simulink library "NCS_Library"  (R2019a)
settings: Solver=VariableStepAuto  StartTime=0.0  StopTime=10.0  RelTol=1e-3
values from neighbouring files (symbols this model uses):
  A = 10    [Parameter.m]
  band = 100000000    [Parameter.m]
  BER = 0    [Parameter.m]
  c = 5000000    [Parameter.m]
  c1 = 4.33    [Parameter.m]
  c2 = 3.16    [Parameter.m]
  CAN2EthernetDelay = 0.000    (= 0)    [Parameter.m]
  cR = 1.5*10^-3    (= 0.0015)    [Parameter.m]
  cw = (cwE * 2 + cwM * (nW_ges-2))/nW_ges    (= 0.1475)    [Parameter.m]
  cwE = 0.35    [Parameter.m]
  cwM = 0.08    [Parameter.m]
  Cycle_Controller = 0    [Parameter.m]
  CyclePLC = 24/1000    (= 0.024)    [Parameter.m]
  d = 800000    [Parameter.m]
  Dr = 0.92    [Parameter.m]
  Ethernet2CANDelay = 0.005    [Parameter.m]
  F_konst = 70892    [Parameter.m]
  FA = 100000    [Parameter.m]
  FB_WB_max = 10000    [Parameter.m]
  FBel_an = iG*nG*F_KZmax*nBan*R_mR/(Dr/2)    (= 28197.4297239)    [Parameter.m]
  FBel_frei = iG*nG*F_KZmax*nBfrei*R_mW/(Dr/2)    (= 29270.6882948)    [Parameter.m]
  Fmaxdyn = 300000    [Parameter.m]
  g = 9.81    [Parameter.m]
  i = 0    [Parameter.m]
  J = 1/2*mA*(Dr/2)^2    (= 158.7)    [Parameter.m]
  k1 = 0.095    [Parameter.m]
  k2 = 9.26/3.6    (= 2.57222222222)    [Parameter.m]
  k3 = 4.63/3.6    (= 1.28611111111)    [Parameter.m]
  mges = 58000    [Parameter.m]
  mu = [mu1 mu2]    [Parameter.m]
  muBel1 = 0.42    [Parameter.m]
  muBel2 = 0.36    [Parameter.m]
  n = 0.001    [Parameter.m]
  n_Mg = 4    [Parameter.m]
  n_WB = 4    [Parameter.m]
  nA = 4    [Parameter.m]
  nBan = 2    [Parameter.m]
  nBfrei = 3    [Parameter.m]
  nM = 4    [Parameter.m]
  nW_an = 4    [Parameter.m]
  P_max = 8200000    [Parameter.m]
  Q = 10    [Parameter.m]
  r_reib = 600    [Parameter.m]
  rho = 1.08    [Parameter.m]
  rhoL = 1.225    [Parameter.m]
  Size = 8    [Parameter.m]
  slip = [s1 s2]    [Parameter.m]
  tol = 0.05    [Parameter.m]
  v00 = 100/3.6    (= 27.7777777778)    [Parameter.m]
  v_grenz = 60/3.6    (= 16.6666666667)    [Parameter.m]
  v_opt = 75/3.6    (= 20.8333333333)    [Parameter.m]
  W_opt = 0.5    [Parameter.m]
  WB = 1    [Parameter.m]
  y_opt = sqrt(W_opt)/((1+sqrt(W_opt))^2+W_opt)    [Parameter.m]
undefined symbols (not defined in the file or in its folder): BUSCapacity, CableLength, controlGate, D_dyn, D_mg, EnableBurst, EnableToF, entity, Entity_out, Gate, Gate_4, Gate_5, Gate_ACK, Gate_copy, Gate_RX, getData, gettime, I_dyn, I_mg, m, magnitude, P_dyn, P_mg, ReadAttributes, readdata, ReadData, ReadSize, sigbuilder_block, Timeout, ToB, ToF, v0, v_d, v_soll
libraries: simulink x176, $bdroot x102
(part 2 of 12)

== system NCS_Library/Network/ETB ==
  note: Devices
  note: Bus
  Burst Device : Subsystem  mask{Address=[111 299], Destination=[ 100 200], Size=100, Port=1, ReplyAddress=[0 0], Subscribe=[0 0; 0 0; 0 0; 0 0; 0 0], msgType=Passive, Tx=0, Timeout=0, SDTv2=Disable, EnableToF=off, ToF=0, EnableBurst=off, ToB=0, n_Burst=1000}
      mask prompts: Size "Packet Size [Byte]"; Port "Destination Port"; ReplyAddress "Reply Address"; Tx "Tx [s]"; Timeout "TRDP Timeout [s]"; EnableToF "Enable Failure"; ToF "Time [s]"; EnableBurst "Enable Burst"; ToB "Time [s]"
      mask help: The burst device transmit a user defined number n of useless entities in the network at a user defined time.
      mask init:
      | msgType = uint8(3);
      | Timeout = inf;
      | EnableToF = 0;
      | Tx = 0;
      | % limit n_Burst to 1
      | if n_Burst < 1
      |     n_Burst = 1;
      | end
      mask TypeOptions Port: 1 | 2 | 3 | 4 | 5 | 6 | 7 | 8 | Multicast
      mask TypeOptions msgType: Pull | Push Continuous | Push Discrete | Passive
      mask Callback msgType:
      | % Control parameter visiblity
      | % Disable Tx dialog, if it is not needed, because of a passive ED,
      | % which only receives.
      | 
      | % Get value
      | Modus = get_param(gcb,'msgType');
      | ToF = get_param(gcb,'EnableToF');
      | ToB = get_param(gcb,'EnableBurst');
      | 
      | 
      | % Set the 'MaskVisibilities' property for each box
      | 
      | On = {'on','on','on','on','on','on','on','on','on','on','on','on','on','on','on'}; % Init
      | 
      | % Disable Tx Dialog, if not needed
      | 
      | if strcmp('Passive',Modus) || strcmp('Push Discrete',Modus)
      |     On{8} = 'off';
      | end
      | 
      | if strcmp('off',ToF)
      |     On{12} = 'off';
      | end
      | 
      | if strcmp('off',ToB)
      |     On{14} = 'off';
      |     On{15} = 'off';
      | end
      | 
      | set_param(gcb,'MaskEnables',On );
      mask TypeOptions SDTv2: Disable | Enable
      mask Callback EnableToF:
      | % Control parameter visiblity
      | % Disable Tx dialog, if it is not needed, because of a passive ED,
      | % which only receives.
      | 
      | % Get value
      | Modus = get_param(gcb,'msgType');
      | ToF = get_param(gcb,'EnableToF');
      | ToB = get_param(gcb,'EnableBurst');
      | 
      | 
      | % Set the 'MaskVisibilities' property for each box
      | 
      | On = {'on','on','on','on','on','on','on','on','on','on','on','on','on','on','on'}; % Init
      | 
      | % Disable Tx Dialog, if not needed
      | 
      | if strcmp('Passive',Modus) || strcmp('Push Discrete',Modus)
      |     On{8} = 'off';
      | end
      | 
      | if strcmp('off',ToF)
      |     On{12} = 'off';
      | end
      | 
      | if strcmp('off',ToB)
      |     On{14} = 'off';
      |     On{15} = 'off';
      | end
      | 
      | set_param(gcb,'MaskEnables',On );
      mask Callback EnableBurst:
      | % Control parameter visiblity
      | % Disable Tx dialog, if it is not needed, because of a passive ED,
      | % which only receives.
      | 
      | % Get value
      | Modus = get_param(gcb,'msgType');
      | ToF = get_param(gcb,'EnableToF');
      | ToB = get_param(gcb,'EnableBurst');
      | 
      | 
      | % Set the 'MaskVisibilities' property for each box
      | 
      | On = {'on','on','on','on','on','on','on','on','on','on','on','on','on','on','on'}; % Init
      | 
      | % Disable Tx Dialog, if not needed
      | 
      | if strcmp('Passive',Modus) || strcmp('Push Discrete',Modus)
      |     On{8} = 'off';
      | end
      | 
      | if strcmp('off',ToF)
      |     On{12} = 'off';
      | end
      | 
      | if strcmp('off',ToB)
      |     On{14} = 'off';
      |     On{15} = 'off';
      | end
      | 
      | set_param(gcb,'MaskEnables',On );
      mask DialogControl Container3 Prompt: Modus
      mask DialogControl Container4 Prompt: SDTv2
      mask DialogControl Container6 Prompt: Interrupts
      mask Display: disp([ 'Burst Device' ]);
  Cable : Subsystem  mask{length=0, Cable=Coaxial}
      mask prompts: length "Cable Length (m)"; Cable "Cable Type"
      mask TypeOptions Cable: Coaxial | Other
  Controller Interface : Subsystem  mask{Address=[111 211], Sensors=[0 0; 0 0; 0 0; 0 0], Actuators=[0 0; 0 0; 0 0; 0 0], Size=11, EnableToF=off, ToF=0, Enable_1=off, msgType_1=Push by Controller, SDTv2_1=Disable, Tx_1=0, Enable_2=off, msgType_2=Push by Controller, SDTv2_2=Disable, Tx_2=0, Enable_3=off, msgType_3=Push by Controller, SDTv2_3=Disable, Tx_3=0, Enable_4=off, msgType_4=Push by Controller, SDTv2_4=Disable, Tx_4=0}
      mask prompts: Size "Packet Size [Byte]"; EnableToF "Failure"; ToF "Time [s]"; Enable_1 "Enable"; msgType_1 "Modus"; SDTv2_1 "SDTv2"; Tx_1 "Tx [ms]"; Enable_2 "Enable"; msgType_2 "Modus"; SDTv2_2 "SDTv2"; Tx_2 "Tx [ms]"; Enable_3 "Enable"; msgType_3 "Modus"; SDTv2_3 "SDTv2"; Tx_3 "Tx [ms]"; Enable_4 "Enable"; msgType_4 "Modus"; SDTv2_4 "SDTv2"; Tx_4 "Tx [ms]"
      mask help: Tx can be set to zero in case of a discrete source
      mask init:
      | % Ensure, that Tx is set to zero in the case of pull.
      | if msgType_1 == 2 || ~Enable_1
      |     Tx_1 = inf;
      | else
      |     % convert [ms] to [s]
      |     Tx_1 = Tx_1/1000;
      | end
      | 
      | if msgType_2 == 2 || ~Enable_2
      |     Tx_2 = inf;
      | else
      |     % convert [ms] to [s]
      |     Tx_2 = Tx_2/1000;
      | end
      | 
      | if msgType_3 == 2 || ~Enable_3
      |     Tx_3 = inf;
      | else
      |     % convert [ms] to [s]
      |     Tx_3 = Tx_3/1000;
      | end
      | 
      | if msgType_4 == 2 || ~Enable_4
      |     Tx_4 = inf;
      | else
      |     % convert [ms] to [s]
      |     Tx_4 = Tx_4/1000;
      | end
      | 
      | % 
      | if ~Enable_1 && ~Enable_2 && ~Enable_3 && ~Enable_4
      |     Actuators = zeros(4,2);
      | end
      mask Callback EnableToF:
      | % Control parameter visiblity
      | 
      | % Get the values of the Modus boxes
      | Enable_1 = get_param(gcb,'Enable_1');
      | Enable_2 = get_param(gcb,'Enable_2');
      | Enable_3 = get_param(gcb,'Enable_3');
      | Enable_4 = get_param(gcb,'Enable_4');
      | 
      | Modus_1 = get_param(gcb,'msgType_1');
      | Modus_2 = get_param(gcb,'msgType_2');
      | Modus_3 = get_param(gcb,'msgType_3');
      | Modus_4 = get_param(gcb,'msgType_4');
      | 
      | EnableToF = get_param(gcb,'EnableToF');
      | 
      | % Set the 'MaskVisibilities' property for each box
      | 
      | On = {'on','on','on','on','on','on','on','on','on','on','on','on','on','on','on','on','on','on','on','on','on','on'}; % Init
      | 
      | % Disable Port Dialog, if not needed
      | if strcmp('off',Enable_1)
      |     On{7} = 'off';
      |     On{8} = 'off';
      |     On{9} = 'off';
      | end
      | if strcmp('off',Enable_2)
      |     On{11} = 'off';
      |     On{12} = 'off';
      |     On{13} = 'off';
      | end
      | if strcmp('off',Enable_3)
      |     On{15} = 'off';
      |     On{16} = 'off';
      |     On{17} = 'off';
      | end
      | if strcmp('off',Enable_4)
      |     On{19} = 'off';
      |     On{20} = 'off';
      |     On{21} = 'off';
      | end
      | 
      | % Disable Tx Dialog, if not needed
      | 
      | if ~strcmp('Push by Controller',Modus_1)
      |     On{9} = 'off';
      | end
      | if ~strcmp('Push by Controller',Modus_2)
      |     On{13} = 'off';
      | end
      | if ~strcmp('Push by Controller',Modus_3)
      |     On{17} = 'off';
      | end
      | if ~strcmp('Push by Controller',Modus_4)
      |     On{21} = 'off';
      | end
      | 
      | if strcmp('off',EnableToF)
      |     On{5} = 'off';
      | end
      | 
      | set_param(gcb,'MaskEnables',On );
      mask Callback Enable_1:
      | % Control parameter visiblity
      | 
      | % Get the values of the Modus boxes
      | Enable_1 = get_param(gcb,'Enable_1');
      | Enable_2 = get_param(gcb,'Enable_2');
      | Enable_3 = get_param(gcb,'Enable_3');
      | Enable_4 = get_param(gcb,'Enable_4');
      | 
      | Modus_1 = get_param(gcb,'msgType_1');
      | Modus_2 = get_param(gcb,'msgType_2');
      | Modus_3 = get_param(gcb,'msgType_3');
      | Modus_4 = get_param(gcb,'msgType_4');
      | 
      | EnableToF = get_param(gcb,'EnableToF');
      | 
      | % Set the 'MaskVisibilities' property for each box
      | 
      | On = {'on','on','on','on','on','on','on','on','on','on','on','on','on','on','on','on','on','on','on','on','on','on'}; % Init
      | 
      | % Disable Port Dialog, if not needed
      | if strcmp('off',Enable_1)
      |     On{7} = 'off';
      |     On{8} = 'off';
      |     On{9} = 'off';
      | end
      | if strcmp('off',Enable_2)
      |     On{11} = 'off';
      |     On{12} = 'off';
      |     On{13} = 'off';
      | end
      | if strcmp('off',Enable_3)
      |     On{15} = 'off';
      |     On{16} = 'off';
      |     On{17} = 'off';
      | end
      | if strcmp('off',Enable_4)
      |     On{19} = 'off';
      |     On{20} = 'off';
      |     On{21} = 'off';
      | end
      | 
      | % Disable Tx Dialog, if not needed
      | 
      | if ~strcmp('Push by Controller',Modus_1)
      |     On{9} = 'off';
      | end
      | if ~strcmp('Push by Controller',Modus_2)
      |     On{13} = 'off';
      | end
      | if ~strcmp('Push by Controller',Modus_3)
      |     On{17} = 'off';
      | end
      | if ~strcmp('Push by Controller',Modus_4)
      |     On{21} = 'off';
      | end
      | 
      | if strcmp('off',EnableToF)
      |     On{5} = 'off';
      | end
      | 
      | set_param(gcb,'MaskEnables',On );
      mask TypeOptions msgType_1: Push by Controller | Pull by Actuator
      mask Callback msgType_1:
      | % Control parameter visiblity
      | 
      | % Get the values of the Modus boxes
      | Enable_1 = get_param(gcb,'Enable_1');
      | Enable_2 = get_param(gcb,'Enable_2');
      | Enable_3 = get_param(gcb,'Enable_3');
      | Enable_4 = get_param(gcb,'Enable_4');
      | 
      | Modus_1 = get_param(gcb,'msgType_1');
      | Modus_2 = get_param(gcb,'msgType_2');
      | Modus_3 = get_param(gcb,'msgType_3');
      | Modus_4 = get_param(gcb,'msgType_4');
      | 
      | EnableToF = get_param(gcb,'EnableToF');
      | 
      | % Set the 'MaskVisibilities' property for each box
      | 
      | On = {'on','on','on','on','on','on','on','on','on','on','on','on','on','on','on','on','on','on','on','on','on','on'}; % Init
      | 
      | % Disable Port Dialog, if not needed
      | if strcmp('off',Enable_1)
      |     On{7} = 'off';
      |     On{8} = 'off';
      |     On{9} = 'off';
      | end
      | if strcmp('off',Enable_2)
      |     On{11} = 'off';
      |     On{12} = 'off';
      |     On{13} = 'off';
      | end
      | if strcmp('off',Enable_3)
      |     On{15} = 'off';
      |     On{16} = 'off';
      |     On{17} = 'off';
      | end
      | if strcmp('off',Enable_4)
      |     On{19} = 'off';
      |     On{20} = 'off';
      |     On{21} = 'off';
      | end
      | 
      | % Disable Tx Dialog, if not needed
      | 
      | if ~strcmp('Push by Controller',Modus_1)
      |     On{9} = 'off';
      | end
      | if ~strcmp('Push by Controller',Modus_2)
      |     On{13} = 'off';
      | end
      | if ~strcmp('Push by Controller',Modus_3)
      |     On{17} = 'off';
      | end
      | if ~strcmp('Push by Controller',Modus_4)
      |     On{21} = 'off';
      | end
      | 
      | if strcmp('off',EnableToF)
      |     On{5} = 'off';
      | end
      | 
      | set_param(gcb,'MaskEnables',On );
      mask TypeOptions SDTv2_1: Disable | Enable
      mask Callback Enable_2:
      | % Control parameter visiblity
      | 
      | % Get the values of the Modus boxes
      | Enable_1 = get_param(gcb,'Enable_1');
      | Enable_2 = get_param(gcb,'Enable_2');
      | Enable_3 = get_param(gcb,'Enable_3');
      | Enable_4 = get_param(gcb,'Enable_4');
      | 
      | Modus_1 = get_param(gcb,'msgType_1');
      | Modus_2 = get_param(gcb,'msgType_2');
      | Modus_3 = get_param(gcb,'msgType_3');
      | Modus_4 = get_param(gcb,'msgType_4');
      | 
      | EnableToF = get_param(gcb,'EnableToF');
      | 
      | % Set the 'MaskVisibilities' property for each box
      | 
      | On = {'on','on','on','on','on','on','on','on','on','on','on','on','on','on','on','on','on','on','on','on','on','on'}; % Init
      | 
      | % Disable Port Dialog, if not needed
      | if strcmp('off',Enable_1)
      |     On{7} = 'off';
      |     On{8} = 'off';
      |     On{9} = 'off';
      | end
      | if strcmp('off',Enable_2)
      |     On{11} = 'off';
      |     On{12} = 'off';
      |     On{13} = 'off';
      | end
      | if strcmp('off',Enable_3)
      |     On{15} = 'off';
      |     On{16} = 'off';
      |     On{17} = 'off';
      | end
      | if strcmp('off',Enable_4)
      |     On{19} = 'off';
      |     On{20} = 'off';
      |     On{21} = 'off';
      | end
      | 
      | % Disable Tx Dialog, if not needed
      | 
      | if ~strcmp('Push by Controller',Modus_1)
      |     On{9} = 'off';
      | end
      | if ~strcmp('Push by Controller',Modus_2)
      |     On{13} = 'off';
      | end
      | if ~strcmp('Push by Controller',Modus_3)
      |     On{17} = 'off';
      | end
      | if ~strcmp('Push by Controller',Modus_4)
      |     On{21} = 'off';
      | end
      | 
      | if strcmp('off',EnableToF)
      |     On{5} = 'off';
      | end
      | 
      | set_param(gcb,'MaskEnables',On );
      mask TypeOptions msgType_2: Push by Controller | Pull by Actuator
      mask Callback msgType_2:
      | % Control parameter visiblity
      | 
      | % Get the values of the Modus boxes
      | Enable_1 = get_param(gcb,'Enable_1');
      | Enable_2 = get_param(gcb,'Enable_2');
      | Enable_3 = get_param(gcb,'Enable_3');
      | Enable_4 = get_param(gcb,'Enable_4');
      | 
      | Modus_1 = get_param(gcb,'msgType_1');
      | Modus_2 = get_param(gcb,'msgType_2');
      | Modus_3 = get_param(gcb,'msgType_3');
      | Modus_4 = get_param(gcb,'msgType_4');
      | 
      | EnableToF = get_param(gcb,'EnableToF');
      | 
      | % Set the 'MaskVisibilities' property for each box
      | 
      | On = {'on','on','on','on','on','on','on','on','on','on','on','on','on','on','on','on','on','on','on','on','on','on'}; % Init
      | 
      | % Disable Port Dialog, if not needed
      | if strcmp('off',Enable_1)
      |     On{7} = 'off';
      |     On{8} = 'off';
      |     On{9} = 'off';
      | end
      | if strcmp('off',Enable_2)
      |     On{11} = 'off';
      |     On{12} = 'off';
      |     On{13} = 'off';
      | end
      | if strcmp('off',Enable_3)
      |     On{15} = 'off';
      |     On{16} = 'off';
      |     On{17} = 'off';
      | end
      | if strcmp('off',Enable_4)
      |     On{19} = 'off';
      |     On{20} = 'off';
      |     On{21} = 'off';
      | end
      | 
      | % Disable Tx Dialog, if not needed
      | 
      | if ~strcmp('Push by Controller',Modus_1)
      |     On{9} = 'off';
      | end
      | if ~strcmp('Push by Controller',Modus_2)
      |     On{13} = 'off';
      | end
      | if ~strcmp('Push by Controller',Modus_3)
      |     On{17} = 'off';
      | end
      | if ~strcmp('Push by Controller',Modus_4)
      |     On{21} = 'off';
      | end
      | 
      | if strcmp('off',EnableToF)
      |     On{5} = 'off';
      | end
      | 
      | set_param(gcb,'MaskEnables',On );
      mask TypeOptions SDTv2_2: Disable | Enable
      mask Callback Enable_3:
      | % Control parameter visiblity
      | 
      | % Get the values of the Modus boxes
      | Enable_1 = get_param(gcb,'Enable_1');
      | Enable_2 = get_param(gcb,'Enable_2');
      | Enable_3 = get_param(gcb,'Enable_3');
      | Enable_4 = get_param(gcb,'Enable_4');
      | 
      | Modus_1 = get_param(gcb,'msgType_1');
      | Modus_2 = get_param(gcb,'msgType_2');
      | Modus_3 = get_param(gcb,'msgType_3');
      | Modus_4 = get_param(gcb,'msgType_4');
      | 
      | EnableToF = get_param(gcb,'EnableToF');
      | 
      | % Set the 'MaskVisibilities' property for each box
      | 
      | On = {'on','on','on','on','on','on','on','on','on','on','on','on','on','on','on','on','on','on','on','on','on','on'}; % Init
      | 
      | % Disable Port Dialog, if not needed
      | if strcmp('off',Enable_1)
      |     On{7} = 'off';
      |     On{8} = 'off';
      |     On{9} = 'off';
      | end
      | if strcmp('off',Enable_2)
      |     On{11} = 'off';
      |     On{12} = 'off';
      |     On{13} = 'off';
      | end
      | if strcmp('off',Enable_3)
      |     On{15} = 'off';
      |     On{16} = 'off';
      |     On{17} = 'off';
      | end
      | if strcmp('off',Enable_4)
      |     On{19} = 'off';
      |     On{20} = 'off';
      |     On{21} = 'off';
      | end
      | 
      | % Disable Tx Dialog, if not needed
      | 
      | if ~strcmp('Push by Controller',Modus_1)
      |     On{9} = 'off';
      | end
      | if ~strcmp('Push by Controller',Modus_2)
      |     On{13} = 'off';
      | end
      | if ~strcmp('Push by Controller',Modus_3)
      |     On{17} = 'off';
      | end
      | if ~strcmp('Push by Controller',Modus_4)
      |     On{21} = 'off';
      | end
      | 
      | if strcmp('off',EnableToF)
      |     On{5} = 'off';
      | end
      | 
      | set_param(gcb,'MaskEnables',On );
      mask TypeOptions msgType_3: Push by Controller | Pull by Actuator
      mask Callback msgType_3:
      | % Control parameter visiblity
      | 
      | % Get the values of the Modus boxes
      | Enable_1 = get_param(gcb,'Enable_1');
      | Enable_2 = get_param(gcb,'Enable_2');
      | Enable_3 = get_param(gcb,'Enable_3');
      | Enable_4 = get_param(gcb,'Enable_4');
      | 
      | Modus_1 = get_param(gcb,'msgType_1');
      | Modus_2 = get_param(gcb,'msgType_2');
      | Modus_3 = get_param(gcb,'msgType_3');
      | Modus_4 = get_param(gcb,'msgType_4');
      | 
      | EnableToF = get_param(gcb,'EnableToF');
      | 
      | % Set the 'MaskVisibilities' property for each box
      | 
      | On = {'on','on','on','on','on','on','on','on','on','on','on','on','on','on','on','on','on','on','on','on','on','on'}; % Init
      | 
      | % Disable Port Dialog, if not needed
      | if strcmp('off',Enable_1)
      |     On{7} = 'off';
      |     On{8} = 'off';
      |     On{9} = 'off';
      | end
      | if strcmp('off',Enable_2)
      |     On{11} = 'off';
      |     On{12} = 'off';
      |     On{13} = 'off';
      | end
      | if strcmp('off',Enable_3)
      |     On{15} = 'off';
      |     On{16} = 'off';
      |     On{17} = 'off';
      | end
      | if strcmp('off',Enable_4)
      |     On{19} = 'off';
      |     On{20} = 'off';
      |     On{21} = 'off';
      | end
      | 
      | % Disable Tx Dialog, if not needed
      | 
      | if ~strcmp('Push by Controller',Modus_1)
      |     On{9} = 'off';
      | end
      | if ~strcmp('Push by Controller',Modus_2)
      |     On{13} = 'off';
      | end
      | if ~strcmp('Push by Controller',Modus_3)
      |     On{17} = 'off';
      | end
      | if ~strcmp('Push by Controller',Modus_4)
      |     On{21} = 'off';
      | end
      | 
      | if strcmp('off',EnableToF)
      |     On{5} = 'off';
      | end
      | 
      | set_param(gcb,'MaskEnables',On );
      mask TypeOptions SDTv2_3: Disable | Enable
      mask Callback Enable_4:
      | % Control parameter visiblity
      | 
      | % Get the values of the Modus boxes
      | Enable_1 = get_param(gcb,'Enable_1');
      | Enable_2 = get_param(gcb,'Enable_2');
      | Enable_3 = get_param(gcb,'Enable_3');
      | Enable_4 = get_param(gcb,'Enable_4');
      | 
      | Modus_1 = get_param(gcb,'msgType_1');
      | Modus_2 = get_param(gcb,'msgType_2');
      | Modus_3 = get_param(gcb,'msgType_3');
      | Modus_4 = get_param(gcb,'msgType_4');
      | 
      | EnableToF = get_param(gcb,'EnableToF');
      | 
      | % Set the 'MaskVisibilities' property for each box
      | 
      | On = {'on','on','on','on','on','on','on','on','on','on','on','on','on','on','on','on','on','on','on','on','on','on'}; % Init
      | 
      | % Disable Port Dialog, if not needed
      | if strcmp('off',Enable_1)
      |     On{7} = 'off';
      |     On{8} = 'off';
      |     On{9} = 'off';
      | end
      | if strcmp('off',Enable_2)
      |     On{11} = 'off';
      |     On{12} = 'off';
      |     On{13} = 'off';
      | end
      | if strcmp('off',Enable_3)
      |     On{15} = 'off';
      |     On{16} = 'off';
      |     On{17} = 'off';
      | end
      | if strcmp('off',Enable_4)
      |     On{19} = 'off';
      |     On{20} = 'off';
      |     On{21} = 'off';
      | end
      | 
      | % Disable Tx Dialog, if not needed
      | 
      | if ~strcmp('Push by Controller',Modus_1)
      |     On{9} = 'off';
      | end
      | if ~strcmp('Push by Controller',Modus_2)
      |     On{13} = 'off';
      | end
      | if ~strcmp('Push by Controller',Modus_3)
      |     On{17} = 'off';
      | end
      | if ~strcmp('Push by Controller',Modus_4)
      |     On{21} = 'off';
      | end
      | 
      | if strcmp('off',EnableToF)
      |     On{5} = 'off';
      | end
      | 
      | set_param(gcb,'MaskEnables',On );
      mask TypeOptions msgType_4: Push by Controller | Pull by Actuator
      mask Callback msgType_4:
      | % Control parameter visiblity
      | 
      | % Get the values of the Modus boxes
      | Enable_1 = get_param(gcb,'Enable_1');
      | Enable_2 = get_param(gcb,'Enable_2');
      | Enable_3 = get_param(gcb,'Enable_3');
      | Enable_4 = get_param(gcb,'Enable_4');
      | 
      | Modus_1 = get_param(gcb,'msgType_1');
      | Modus_2 = get_param(gcb,'msgType_2');
      | Modus_3 = get_param(gcb,'msgType_3');
      | Modus_4 = get_param(gcb,'msgType_4');
      | 
      | EnableToF = get_param(gcb,'EnableToF');
      | 
      | % Set the 'MaskVisibilities' property for each box
      | 
      | On = {'on','on','on','on','on','on','on','on','on','on','on','on','on','on','on','on','on','on','on','on','on','on'}; % Init
      | 
      | % Disable Port Dialog, if not needed
      | if strcmp('off',Enable_1)
      |     On{7} = 'off';
      |     On{8} = 'off';
      |     On{9} = 'off';
      | end
      | if strcmp('off',Enable_2)
      |     On{11} = 'off';
      |     On{12} = 'off';
      |     On{13} = 'off';
      | end
      | if strcmp('off',Enable_3)
      |     On{15} = 'off';
      |     On{16} = 'off';
      |     On{17} = 'off';
      | end
      | if strcmp('off',Enable_4)
      |     On{19} = 'off';
      |     On{20} = 'off';
      |     On{21} = 'off';
      | end
      | 
      | % Disable Tx Dialog, if not needed
      | 
      | if ~strcmp('Push by Controller',Modus_1)
      |     On{9} = 'off';
      | end
      | if ~strcmp('Push by Controller',Modus_2)
      |     On{13} = 'off';
      | end
      | if ~strcmp('Push by Controller',Modus_3)
      |     On{17} = 'off';
      | end
      | if ~strcmp('Push by Controller',Modus_4)
      |     On{21} = 'off';
      | end
      | 
      | if strcmp('off',EnableToF)
      |     On{5} = 'off';
      | end
      | 
      | set_param(gcb,'MaskEnables',On );
      mask TypeOptions SDTv2_4: Disable | Enable
      mask DialogControl Container13 Prompt: Interrupt
      mask DialogControl Container9 Prompt: Port 1
      mask DialogControl Container10 Prompt: Port 2
      mask DialogControl Container11 Prompt: Port 3
      mask DialogControl Container12 Prompt: Port 4
      mask Display: disp([ 'Ethernet \n Controller Interface' '\n' get_param(gcb,'Address') ]);
  ED : Subsystem  mask{Address=[111 211], Destination=[ 0 0], Port=1, ReplyAddress=[0 0], Size=11, Subscribe=[0 0; 0 0; 0 0; 0 0; 0 0], msgType=Passive, Tx=0, Timeout=2, SDTv2=Disable, EnableToF=off, ToF=0}
      mask prompts: Port "Destination Port"; ReplyAddress "Reply Address"; Size "Packet Size [Byte]"; Tx "Tx [ms]"; Timeout "TRDP Timeout [s]"; EnableToF "Enable Failure"; ToF "Time [s]"
      mask init:
      | if msgType == 3 || msgType == 4
      |     Tx = 0;
      | else
      |     Tx = Tx/1000;
      | end
      mask TypeOptions Port: 1 | 2 | 3 | 4 | 5 | 6 | 7 | 8 | Multicast
      mask TypeOptions msgType: Pull | Push cyclical | Push sporadic | Passive
      mask Callback msgType:
      | % Control parameter visiblity
      | % Disable Tx dialog, if it is not needed, because of a passive ED,
      | % which only receives.
      | 
      | % Get value
      | Modus = get_param(gcb,'msgType');
      | ToF = get_param(gcb,'EnableToF');
      | 
      | % Set the 'MaskVisibilities' property for each box
      | 
      | On = {'on','on','on','on','on','on','on','on','on','on','on','on'}; % Init
      | 
      | % Disable Tx Dialog, if not needed
      | 
      | if strcmp('Passive',Modus) || strcmp('Push Discrete',Modus)
      |     On{8} = 'off';
      | end
      | 
      | if strcmp('off',ToF)
      |     On{12} = 'off';
      | end
      | 
      | set_param(gcb,'MaskEnables',On );
      mask TypeOptions SDTv2: Disable | Enable
      mask Callback EnableToF:
      | % Control parameter visiblity
      | % Disable Tx dialog, if it is not needed, because of a passive ED,
      | % which only receives.
      | 
      | % Get value
      | Modus = get_param(gcb,'msgType');
      | ToF = get_param(gcb,'EnableToF');
      | 
      | % Set the 'MaskVisibilities' property for each box
      | 
      | On = {'on','on','on','on','on','on','on','on','on','on','on','on'}; % Init
      | 
      | % Disable Tx Dialog, if not needed
      | 
      | if strcmp('Passive',Modus) || strcmp('Push Discrete',Modus)
      |     On{8} = 'off';
      | end
      | 
      | if strcmp('off',ToF)
      |     On{12} = 'off';
      | end
      | 
      | set_param(gcb,'MaskEnables',On );
      mask DialogControl Container3 Prompt: Modus
      mask DialogControl Container4 Prompt: SDTv2
      mask DialogControl Container6 Prompt: Interrupts
      mask Display: disp([ 'End Device' '\n' get_param(gcb,'Address') ]);
  Ethernet_2-port_Switch : Subsystem  mask{addstore=10, bandc=10^8, buffer_size=120000, cable_node=0, cable_LR=0}
      mask prompts: addstore "Number of Addresses to Store on each Port"; bandc "Bandwidth for Switch [bits/s]"; buffer_size "Total Buffer size [bits]"; cable_node "Length of Cable to Node [m]"; cable_LR "Length of Cable to L or R [m]"
      mask init:
      | % band = eval(band);
      mask TypeOptions bandc: 10^7 | 10^8 | 10^9
      mask DialogControl DescGroupVar Prompt: Ethernet 2-Port Switch
      mask DialogControl DescTextVar Prompt: Ethernet Switch with Two Ports, for use at the end of the network.
  Ethernet_3-port_switch : Subsystem  mask{addstore=5, bandc=10^8, buffer_size=180000, cable_node=0, cable_L=0, cable_R=0}
      mask prompts: addstore "Number of addresses to Store on each port"; bandc "Bandwidth of switch [bits/s]"; buffer_size "Total Buffer Size [bits]"; cable_node "Cable length to Node"; cable_L "Cable length to L"; cable_R "Cable length to R"
      mask init:
      | %band = eval(band);
      mask TypeOptions bandc: 10^7 | 10^8 | 10^9
      mask DialogControl DescGroupVar Prompt: Ethernet Switch 3 Ports
      mask DialogControl DescTextVar Prompt: Ethernet Switch with 3 Ports, for use between other switches or nodes within a network.
  OSI Layers : Subsystem
  Subsystem2 : Subsystem  mask{RouterID=1, SubnetIDa=0, SubnetIDb=0, SubnetIDc=0, CycleTime_Router=0.05, EnableToF=off, ToF=0}
      mask prompts: SubnetIDa "1. Subnet"; SubnetIDb "2. Subnet"; SubnetIDc "3. Subnet"; CycleTime_Router "CycleTime"; EnableToF "Failure"; ToF "Time of Failure [s]"
      mask Callback EnableToF:
      | % Control parameter visiblity
      | 
      | % Get value
      | ToF = get_param(gcb,'EnableToF');
      | 
      | 
      | % Set the 'MaskVisibilities' property for each box
      | 
      | On = {'on','on','on','on','on','on','on'}; % Init
      | 
      | % Disable Time Dialog, if not needed
      | if strcmp('off',ToF)
      |     On{7} = 'off';
      | end
      | 
      | set_param(gcb,'MaskEnables',On );
      mask DialogControl Container4 Prompt: Interrupt
      mask Display: disp([ 'Router' '\n ID: '  get_param(gcb,'RouterID') ]);
  Termination : Subsystem

== system NCS_Library/Network/Gateway ==
  note: CAN 1
  note: CAN 2
  Gateway1 : Subsystem  mask{T_Tx=4, MaxNum=20, Address=[111 211], Destination=[0 0], Port=1, ReplyAddress=[0 0], Subscribe=[0 0; 0 0; 0 0; 0 0; 0 0], Timeout=inf, SDTv2=Disable, SensorType=0, MsgID=25, IDRange=[1:25], T_Tx_CAN=0.1, MsgSize=8, IDSubscription=[0,0,0,0,0,0,0,0,0,0,0,0,0,0,0,0,0,0,0,0,0,0,0,0,0], EnableToF=off, ToF=0}
      mask prompts: Port "Destination Port"; ReplyAddress "Reply Address"; MsgID "CAN ID"; IDRange "Range of all IDs"; T_Tx_CAN "T_Tx"; MsgSize "DataSIze (0-8 Bytes)"; IDSubscription "IDs of messages subscribed to accept (0-no, 1-yes)"; EnableToF "Failure"; ToF "Time [s]"
      mask TypeOptions Port: 1 | 2 | 3 | 4 | 5 | 6 | 7 | 8 | Multicast
      mask TypeOptions SDTv2: Disable | Enable
      mask Callback EnableToF:
      | % Control parameter visiblity
      | % Disable Tx dialog, if it is not needed, because of a passive ED,
      | % which only receives.
      | 
      | % Get value
      | ToF = get_param(gcb,'EnableToF');
      | % ToB = get_param(gcb,'EnableBurst');
      | 
      | 
      | % Set the 'MaskVisibilities' property for each box
      | 
      | On = {'on','on','on','on','on','on','on','on','on','on','on','on','on','on','on','on','on'}; % Init
      | 
      | % Disable Tx Dialog, if not needed
      | if strcmp('off',ToF)
      |     On{17} = 'off';
      | end
      | 
      | set_param(gcb,'MaskEnables',On );
      mask DialogControl ParameterGroupVar Prompt: Parameters Gateway
      mask DialogControl Container5 Prompt: Parameters Ethernet Interface
      mask DialogControl Container6 Prompt: SDTv2
      mask DialogControl Container3 Prompt: Paramters CAN Interface
      mask DialogControl Container4 Prompt: Interupts
      mask Display: disp( ['Address: ', get_param(gcb,'Address'), '\n \n Ethernet-CAN-Gateway', '\n \n CAN-ID: ', get_param(gcb,'msgID')] )
  Gateway2 : Subsystem  mask{T_Tx=4, MaxNum=20, Address=[111 211], Destination=[0 0], Port=1, ReplyAddress=[0 0], Subscribe=[0 0; 0 0; 0 0; 0 0; 0 0], Timeout=inf, SDTv2=Disable, SensorType=0, MsgID=25, IDRange=[1:25], T_Tx_CAN=0.1, MsgSize=8, IDSubscription=[0,0,0,0,0,0,0,0,0,0,0,0,0,0,0,0,0,0,0,0,0,0,0,0,0], EnableToF=off, ToF=0}
      mask prompts: Port "Destination Port"; ReplyAddress "Reply Address"; MsgID "CAN ID"; IDRange "Range of all IDs"; T_Tx_CAN "T_Tx"; MsgSize "DataSIze (0-8 Bytes)"; IDSubscription "IDs of messages subscribed to accept (0-no, 1-yes)"; EnableToF "Failure"; ToF "Time [s]"
      mask TypeOptions Port: 1 | 2 | 3 | 4 | 5 | 6 | 7 | 8 | Multicast
      mask TypeOptions SDTv2: Disable | Enable
      mask Callback EnableToF:
      | % Control parameter visiblity
      | % Disable Tx dialog, if it is not needed, because of a passive ED,
      | % which only receives.
      | 
      | % Get value
      | ToF = get_param(gcb,'EnableToF');
      | % ToB = get_param(gcb,'EnableBurst');
      | 
      | 
      | % Set the 'MaskVisibilities' property for each box
      | 
      | On = {'on','on','on','on','on','on','on','on','on','on','on','on','on','on','on','on','on'}; % Init
      | 
      | % Disable Tx Dialog, if not needed
      | if strcmp('off',ToF)
      |     On{17} = 'off';
      | end
      | 
      | set_param(gcb,'MaskEnables',On );
      mask DialogControl ParameterGroupVar Prompt: Parameters Gateway
      mask DialogControl Container5 Prompt: Parameters Ethernet Interface
      mask DialogControl Container6 Prompt: SDTv2
      mask DialogControl Container3 Prompt: Paramters CAN Interface
      mask DialogControl Container4 Prompt: Interupts
      mask Display: disp( ['Address: ', get_param(gcb,'Address'), '\n \n Ethernet-CAN-Gateway', '\n \n CAN-ID: ', get_param(gcb,'msgID')] )

== system NCS_Library/Plant (Train)/Angetriebene_Achse ==
  note: Elektromotor
  note: F_t
  note: Schlupf
  fSt_dyn : Inport
  fSt Achse : Inport  Port=2
  Wagengeschwindigkeit : Inport  Port=3
  1/I : Gain  Gain=1/J  SaturateOnIntegerOverflow=on  OutDataTypeStr=Inherit: Same as input  ParamDataTypeStr=Inherit: Same as input
  Add : Sum  Inputs=-+
  Bremskraft pro angetriebener Achse2 : Subsystem
  Bus Creator : BusCreator  Inputs=3
  Display{,1..6} (7 alike) : Display
  Gain : Gain  Gain=1/1000
  Gain1 : Gain  Gain=1/(Dr/2)  SaturateOnIntegerOverflow=on  OutDataTypeStr=Inherit: Same as input  ParamDataTypeStr=Inherit: Same as input
  Gain2 : Gain
  Kraftschlussbeiwert : Scope
  Max : MinMax  Function=max  Inputs=2
  Neigung : Constant  Value=i
  Product : Product  Inputs=3
  Rad- geschwindigkeit : Integrator  InitialCondition=v0/(Dr/2)  LimitOutput=on  UpperSaturationLimit=1000  LowerSaturationLimit=0
  Radradius : Gain  Gain=Dr/2  SaturateOnIntegerOverflow=on  OutDataTypeStr=Inherit: Same as input  ParamDataTypeStr=Inherit: Same as input
  Radradius1 : Gain  Gain=Dr/2  SaturateOnIntegerOverflow=on  OutDataTypeStr=Inherit: Same as input  ParamDataTypeStr=Inherit: Same as input
  Radradius2 : Gain  Gain=Dr/2  SaturateOnIntegerOverflow=on  OutDataTypeStr=Inherit: Same as input  ParamDataTypeStr=Inherit: Same as input
  Schlupf : Fcn  Expr=abs(u(2)-u(1))/u(3)
  Schlupf-Kraftschluss- Beziehung : Lookup_n-D  NumberOfTableDimensions=1  BreakpointsForDimension1=slip  Table=mu  RndMeth=Simplest  SaturateOnIntegerOverflow=on  InputSameDT=on
  Sign : Signum
  Subtract : Sum  Inputs=-+
  Sum1 : Sum  Inputs=--  SaturateOnIntegerOverflow=on  InputSameDT=on  OutDataTypeStr=Inherit: Same as first input
  Trigonometric Function : Trigonometry  Operator=atan
  Trigonometric Function1 : Trigonometry  Operator=cos
  Weight : Gain  Gain=(mges/4)*g  SaturateOnIntegerOverflow=on  OutDataTypeStr=Inherit: Same as input  ParamDataTypeStr=Inherit: Same as input
  cR : Constant  Value=cR
  F_t : Outport
  wires:
  Radradius1/1 -> Display4/1, Bremskraft pro angetriebener Achse2/1(v)  "v"
  Bremskraft pro angetriebener Achse2/1(F_B,A) -> Radradius/1
  Radradius/1 -> Display3/1, Sum1/1
  fSt Achse/1 -> Bremskraft pro angetriebener Achse2/3(f_St_pneumatic)
  fSt_dyn/1 -> Bremskraft pro angetriebener Achse2/2(f_St,dyn)
  Schlupf-Kraftschluss- Beziehung/1 -> Kraftschlussbeiwert/1, Add/1  "mu(s_x)"
  Radradius2/1 -> Sum1/2, Display2/1  "M_t"
  Gain/1 -> Trigonometric Function/1
  cR/1 -> Add/2
  Trigonometric Function/1 -> Trigonometric Function1/1  "phi"
  Trigonometric Function1/1 -> Weight/1
  Neigung/1 -> Gain/1
  Add/1 -> Product/2
  Weight/1 -> Product/1  "F_N"
  Product/1 -> Radradius2/1, F_t/1  "F_t"
  Rad- geschwindigkeit/1 -> Max/2, Subtract/1, Display6/1, Bus Creator/1, Radradius1/1  "omega"
  Bus Creator/1 -> Schlupf/1
  Schlupf/1 -> Display/1, Schlupf-Kraftschluss- Beziehung/1  "s_x"
  1/I/1 -> Rad- geschwindigkeit/1  "dot_omega"
  Sign/1 -> Display1/1, Gain2/1  "sgn(v_s)"
  Subtract/1 -> Sign/1  "v_s"
  Wagengeschwindigkeit/1 -> Gain1/1  "v"
  Sum1/1 -> 1/I/1
  Max/1 -> Bus Creator/3
  Gain1/1 -> Subtract/2, Max/1, Display5/1, Bus Creator/2  "omega_0"
  Gain2/1 -> Product/3

== system NCS_Library/Plant (Train)/Freie_Achse ==
  note: Schlupf
  note: Schlupf
  note: Break
  fSt Achse 1 : Inport
  Wagengeschwindigkeit : Inport  Port=2
  1/I : Gain  Gain=1/J  SaturateOnIntegerOverflow=on  OutDataTypeStr=Inherit: Same as input  ParamDataTypeStr=Inherit: Same as input
  Add : Sum  Inputs=-+
  Bremskraft pro freier Achse1 : Subsystem
  Bus Creator : BusCreator  Inputs=3
  Display : Display
  Display1 : Display
  Gain : Gain  Gain=1/1000
  Gain2 : Gain  Gain=1/(Dr/2)  SaturateOnIntegerOverflow=on  OutDataTypeStr=Inherit: Same as input  ParamDataTypeStr=Inherit: Same as input
  Kraftschlussbeiwert : Scope
  Max : MinMax  Function=max  Inputs=2
  Neigung : Constant  Value=i
  Product : Product  Inputs=3
  Rad- geschwindigkeit : Integrator  InitialCondition=v0/(Dr/2)  LimitOutput=on  UpperSaturationLimit=1000  LowerSaturationLimit=0
  Radgeschwindigkeit : Scope
  Radradius : Gain  Gain=Dr/2  SaturateOnIntegerOverflow=on  OutDataTypeStr=Inherit: Same as input  ParamDataTypeStr=Inherit: Same as input
  Radradius1 : Gain  Gain=Dr/2  SaturateOnIntegerOverflow=on  OutDataTypeStr=Inherit: Same as input  ParamDataTypeStr=Inherit: Same as input
  Radradius2 : Gain  Gain=Dr/2  SaturateOnIntegerOverflow=on  OutDataTypeStr=Inherit: Same as input  ParamDataTypeStr=Inherit: Same as input
  Schlupf : Fcn  Expr=abs(u(2)-u(1))/u(3)
  Schlupf-Kraftschluss- Beziehung : Lookup_n-D  NumberOfTableDimensions=1  BreakpointsForDimension1=slip  Table=mu  RndMeth=Simplest  SaturateOnIntegerOverflow=on  InputSameDT=on
  Schlupfdiagramm : Scope
  Sign : Signum
  Subtract : Sum  Inputs=-+
  Sum1 : Sum  Inputs=--  SaturateOnIntegerOverflow=on  InputSameDT=on  OutDataTypeStr=Inherit: Same as first input
  Trigonometric Function : Trigonometry  Operator=atan
  Trigonometric Function1 : Trigonometry  Operator=cos
  Weight : Gain  Gain=(mges/4)*g  SaturateOnIntegerOverflow=on  OutDataTypeStr=Inherit: Same as input  ParamDataTypeStr=Inherit: Same as input
  cR : Constant  Value=cR
  F_t : Outport
  wires:
  Trigonometric Function1/1 -> Weight/1
  Add/1 -> Product/2
  Gain/1 -> Trigonometric Function/1
  Trigonometric Function/1 -> Trigonometric Function1/1  "phi"
  Neigung/1 -> Gain/1
  Wagengeschwindigkeit/1 -> Gain2/1  "v"
  Sum1/1 -> 1/I/1
  1/I/1 -> Rad- geschwindigkeit/1  "dot_omega"
  Radradius/1 -> Display/1, Sum1/1  "M_B"
  Rad- geschwindigkeit/1 -> Max/2, Subtract/1, Bus Creator/1, Radgeschwindigkeit/1, Radradius1/1  "omega"
  Bremskraft pro freier Achse1/1(F_B) -> Radradius/1  "F_B"
  Radradius2/1 -> Sum1/2  "M_t"
  Schlupf-Kraftschluss- Beziehung/1 -> Kraftschlussbeiwert/1, Add/1  "mu(s_x)"
  Bus Creator/1 -> Schlupf/1
  Product/1 -> Radradius2/1, F_t/1  "F_t"
  Radradius1/1 -> Bremskraft pro freier Achse1/1(v)
  Subtract/1 -> Sign/1  "v_s"
  Sign/1 -> Product/3  "sgn(v_s)"
  Schlupf/1 -> Schlupfdiagramm/1, Schlupf-Kraftschluss- Beziehung/1  "s_x"
  fSt Achse 1/1 -> Bremskraft pro freier Achse1/2(fSt Achse 1)
  Gain2/1 -> Bus Creator/2, Subtract/2, Max/1
  cR/1 -> Add/2
  Max/1 -> Bus Creator/3
  Weight/1 -> Display1/1, Product/1  "F_N"

== system NCS_Library/Plant (Train)/Kupplung ==
  v_vorne : Inport
  x_vorne : Inport  Port=2
  v_hinten : Inport  Port=3
  x_hinten : Inport  Port=4
  Add : Sum
  Dämpferkraft1-2 : Subsystem
      mask Display: image('dämper.png');
  Federkraft1-2 : Subsystem
      mask Display: image('feder.png');
  übertragene Kraft : Outport
  wires:
  v_hinten/1 -> Dämpferkraft1-2/2(v2)
  v_vorne/1 -> Dämpferkraft1-2/1(v1)
  x_hinten/1 -> Federkraft1-2/2(s2)
  x_vorne/1 -> Federkraft1-2/1(s1)
  Federkraft1-2/1(Ff1-2) -> Add/1
  Dämpferkraft1-2/1(Fd1-2) -> Add/2
  Add/1 -> übertragene Kraft/1

== system NCS_Library/Plant (Train)/Stellglied ==
  u : Inport
  Bremskraftaufbau_Schiene1 : TransferFcn  Numerator=[3]  Denominator=[1.5 3]
  Demux : Demux  Outputs=3
  Kraftaufbau_Motor1 : TransferFcn  Denominator=[0.1 1]
  Kraftaufbau_Pneumatik3 : TransferFcn  Numerator=[3]  Denominator=[3 3]
  Mux1 : Mux  Inputs=3
  u_s : Outport
  wires:
  Demux/1 -> Kraftaufbau_Pneumatik3/1  "fSt_Achse"
  Mux1/1 -> u_s/1
  u/1 -> Demux/1
  Demux/3 -> Bremskraftaufbau_Schiene1/1
  Kraftaufbau_Pneumatik3/1 -> Mux1/1
  Kraftaufbau_Motor1/1 -> Mux1/2
  Bremskraftaufbau_Schiene1/1 -> Mux1/3
  Demux/2 -> Kraftaufbau_Motor1/1

== system NCS_Library/Plant (Train)/angetriebener Endwagen ==
  F_vorne : Inport
  fSt Achse 1 : Inport  Port=2
  fSt Achse 2 : Inport  Port=3
  fSt Achse 3 : Inport  Port=4
  fSt Achse 4 : Inport  Port=5
  fSt_dyn : Inport  Port=6
  F_hinten : Inport  Port=7
  Add : Sum  Inputs=++++
  Angetriebene_Achse{1..4} (4 alike) : $bdroot/Plant (Train)/Angetriebene_Achse  SystemSampleTime=-1
  angetriebener Wagen : $bdroot/Plant (Train)/angetriebener Wagen  SystemSampleTime=-1
  s : Outport
  v : Outport  Port=2
  a : Outport  Port=3
  wires:
  F_vorne/1 -> angetriebener Wagen/2
  F_hinten/1 -> angetriebener Wagen/3
  angetriebener Wagen/2 -> a/1
  angetriebener Wagen/3 -> s/1
  angetriebener Wagen/1 -> v/1, Angetriebene_Achse4/3, Angetriebene_Achse3/3, Angetriebene_Achse2/3, Angetriebene_Achse1/3
  Add/1 -> angetriebener Wagen/1
  fSt Achse 1/1 -> Angetriebene_Achse1/2
  fSt Achse 2/1 -> Angetriebene_Achse2/2
  fSt Achse 3/1 -> Angetriebene_Achse3/2
  fSt Achse 4/1 -> Angetriebene_Achse4/2
  fSt_dyn/1 -> Angetriebene_Achse4/1, Angetriebene_Achse3/1, Angetriebene_Achse2/1, Angetriebene_Achse1/1
  Angetriebene_Achse1/1 -> Add/1
  Angetriebene_Achse2/1 -> Add/2
  Angetriebene_Achse3/1 -> Add/3
  Angetriebene_Achse4/1 -> Add/4

== system NCS_Library/Plant (Train)/angetriebener Endwagen Merz ==
  F_vorne : Inport
  fSt Achse 1 : Inport  Port=2
  fSt Achse 2 : Inport  Port=3
  fSt Achse 3 : Inport  Port=4
  fSt Achse 4 : Inport  Port=5
  fSt_dyn : Inport  Port=6
  F_hinten : Inport  Port=7
  Achse_1 : Subsystem
  Achse_2 : Subsystem
  Achse_3 : Subsystem
  Achse_4 : Subsystem
  Add : Sum  Inputs=++++
  Wagen : Subsystem
  s : Outport
  v : Outport  Port=2
  a : Outport  Port=3
  wires:
  F_vorne/1 -> Wagen/2(F_vorne)
  F_hinten/1 -> Wagen/3(F_hinten)
  Wagen/2(a) -> a/1
  Wagen/3(s) -> s/1
  Wagen/1(v) -> v/1, Achse_2/3(Wagengeschwindigkeit), Achse_1/3(Wagengeschwindigkeit), Achse_3/3(Wagengeschwindigkeit), Achse_4/3(Wagengeschwindigkeit)
  Add/1 -> Wagen/1(mu-abhängige Kraft)
  fSt Achse 1/1 -> Achse_1/2(fSt Achse 1)
  fSt Achse 2/1 -> Achse_2/2(fSt Achse 2)
  fSt Achse 3/1 -> Achse_3/2(fSt Achse 3)
  fSt Achse 4/1 -> Achse_4/2(fSt Achse 4)
  fSt_dyn/1 -> Achse_2/1(fSt_dyn), Achse_1/1(fSt_dyn), Achse_3/1(fSt_dyn), Achse_4/1(fSt_dyn)
  Achse_1/1(Tangentialkraft_A1) -> Add/1
  Achse_2/1(Tangentialkraft_A2) -> Add/2
  Achse_3/1(Tangentialkraft_A3) -> Add/3
  Achse_4/1(Tangentialkraft_A4) -> Add/4

== system NCS_Library/Plant (Train)/angetriebener Mittelwagen ==
  F_vorne : Inport
  fSt Achse 1 : Inport  Port=2
  fSt Achse 2 : Inport  Port=3
  fSt Achse 3 : Inport  Port=4
  fSt Achse 4 : Inport  Port=5
  fSt_dyn : Inport  Port=6
  F_hinten : Inport  Port=7
  Add : Sum  Inputs=++++
  Angetriebene_Achse{1..4} (4 alike) : $bdroot/Plant (Train)/Angetriebene_Achse  SystemSampleTime=-1
  angetriebener Wagen : $bdroot/Plant (Train)/angetriebener Wagen  SystemSampleTime=-1
  s : Outport
  v : Outport  Port=2
  a : Outport  Port=3
  wires:
  fSt_dyn/1 -> Angetriebene_Achse4/1, Angetriebene_Achse3/1, Angetriebene_Achse2/1, Angetriebene_Achse1/1
  fSt Achse 4/1 -> Angetriebene_Achse4/2
  fSt Achse 3/1 -> Angetriebene_Achse3/2
  fSt Achse 2/1 -> Angetriebene_Achse2/2
  fSt Achse 1/1 -> Angetriebene_Achse1/2
  Add/1 -> angetriebener Wagen/1
  angetriebener Wagen/1 -> v/1, Angetriebene_Achse4/3, Angetriebene_Achse3/3, Angetriebene_Achse2/3, Angetriebene_Achse1/3
  angetriebener Wagen/3 -> s/1
  angetriebener Wagen/2 -> a/1
  F_hinten/1 -> angetriebener Wagen/3
  F_vorne/1 -> angetriebener Wagen/2
  Angetriebene_Achse2/1 -> Add/2
  Angetriebene_Achse3/1 -> Add/3
  Angetriebene_Achse4/1 -> Add/4
  Angetriebene_Achse1/1 -> Add/1

== system NCS_Library/Plant (Train)/angetriebener Wagen ==
  mu-abhängige Kraft : Inport
  F_vorne : Inport  Port=2
  F_hinten : Inport  Port=3
  Add : Sum  Inputs=++--
  Display{,1..3} (4 alike) : Display
  Divide : Product  Inputs=*/
  Fahrwiderstand_Wagen : Subsystem
  Integrator : Integrator  InitialCondition=v0  LimitOutput=on  LowerSaturationLimit=tol  ShowSaturationPort=on
  Integrator1 : Integrator
  Neigung : Constant  Value=i
  Scope : Scope
  Stop Simulation : Stop
  Wagenmasse : Constant  Value=mges
  rho : Gain  Gain=rho
  v : Outport
  a : Outport  Port=2
  s : Outport  Port=3
  wires:
  rho/1 -> Divide/2
  Add/1 -> Divide/1
  Integrator1/1 -> s/1
  Neigung/1 -> Fahrwiderstand_Wagen/2(Neigung in Promille)
  Wagenmasse/1 -> rho/1, Fahrwiderstand_Wagen/3(mges)
  F_vorne/1 -> Display2/1, Add/2
  Integrator/1 -> Integrator1/1, v/1, Fahrwiderstand_Wagen/1(v)
  F_hinten/1 -> Display3/1, Add/3
  Divide/1 -> Integrator/1, a/1
  Integrator/2 -> Scope/1
  mu-abhängige Kraft/1 -> Display/1, Add/1
  Fahrwiderstand_Wagen/1(Fw) -> Display1/1, Add/4

== system NCS_Library/Plant (Train)/freier Endwagen ==
  F_vorne : Inport
  fSt Achse 1 : Inport  Port=2
  fSt Achse 2 : Inport  Port=3
  fSt Achse 3 : Inport  Port=4
  fSt Achse 4 : Inport  Port=5
  fSt_WB : Inport  Port=6
  F_hinten : Inport  Port=7
  Add : Sum  Inputs=++++
  Freie_Achse{1..4} (4 alike) : $bdroot/Plant (Train)/Freie_Achse  SystemSampleTime=-1
  freier Wagen : $bdroot/Plant (Train)/freier Wagen  SystemSampleTime=-1
  s : Outport
  v : Outport  Port=2
  a : Outport  Port=3
  wires:
  fSt_WB/1 -> freier Wagen/4
  fSt Achse 4/1 -> Freie_Achse4/1
  fSt Achse 3/1 -> Freie_Achse3/1
  fSt Achse 2/1 -> Freie_Achse2/1
  fSt Achse 1/1 -> Freie_Achse1/1
  F_vorne/1 -> freier Wagen/2
  F_hinten/1 -> freier Wagen/3
  freier Wagen/2 -> a/1
  freier Wagen/3 -> s/1
  freier Wagen/1 -> Freie_Achse4/2, Freie_Achse3/2, Freie_Achse2/2, Freie_Achse1/2, v/1
  Freie_Achse2/1 -> Add/2
  Freie_Achse3/1 -> Add/3
  Freie_Achse4/1 -> Add/4
  Add/1 -> freier Wagen/1
  Freie_Achse1/1 -> Add/1

== system NCS_Library/Plant (Train)/freier Mittelwagen ==
  F_vorne : Inport
  fSt Achse 1 : Inport  Port=2
  fSt Achse 2 : Inport  Port=3
  fSt Achse 3 : Inport  Port=4
  fSt Achse 4 : Inport  Port=5
  fSt_WB : Inport  Port=6
  F_hinten : Inport  Port=7
  Add : Sum  Inputs=++++
  Freie_Achse{1..4} (4 alike) : $bdroot/Plant (Train)/Freie_Achse  SystemSampleTime=-1
  freier Wagen : $bdroot/Plant (Train)/freier Wagen  SystemSampleTime=-1
  s : Outport
  v : Outport  Port=2
  a : Outport  Port=3
  wires:
  freier Wagen/1 -> v/1, Freie_Achse4/2, Freie_Achse3/2, Freie_Achse2/2, Freie_Achse1/2
  freier Wagen/3 -> s/1
  freier Wagen/2 -> a/1
  F_hinten/1 -> freier Wagen/3
  F_vorne/1 -> freier Wagen/2
  fSt Achse 1/1 -> Freie_Achse1/1
  fSt Achse 2/1 -> Freie_Achse2/1
  fSt Achse 3/1 -> Freie_Achse3/1
  fSt Achse 4/1 -> Freie_Achse4/1
  fSt_WB/1 -> freier Wagen/4
  Freie_Achse2/1 -> Add/2
  Freie_Achse3/1 -> Add/3
  Freie_Achse4/1 -> Add/4
  Add/1 -> freier Wagen/1
  Freie_Achse1/1 -> Add/1
